simulink model "first"  (R2023b)
settings: Solver=FixedStepAuto  StartTime=0.0  StopTime=10  FixedStep=0.001  RelTol=1e-3
undefined symbols (not defined in the file): A1, A2, B, B2, C2, D2, K1, K2, w0, x0
settings Model: Creator=evdokiiagalkina  LastModifiedBy=evdokiiagalkina

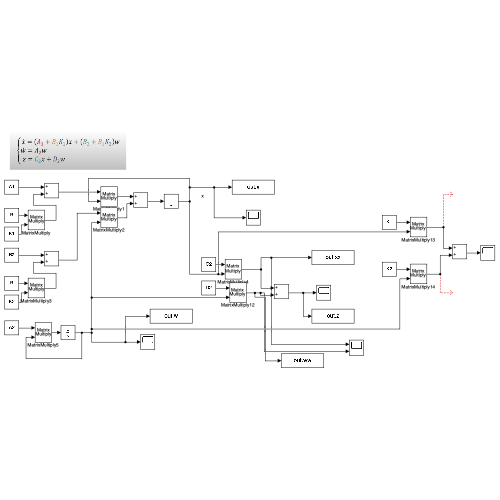
[thumbnail: Simulink's stored preview of the top-level diagram]
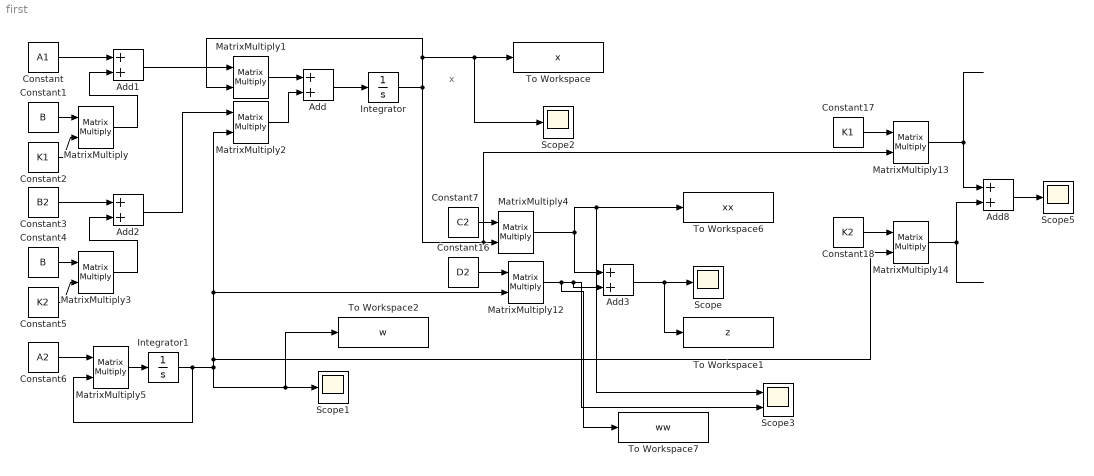
== system first ==
  note: x
  Add{,1..3,8} (5 alike) : Sum
  Constant : Constant  Value=A1  VectorParams1D=off
  Constant1 : Constant  Value=B  VectorParams1D=off
  Constant16 : Constant  Value=D2  VectorParams1D=off
  Constant17 : Constant  Value=K1  VectorParams1D=off
  Constant18 : Constant  Value=K2  VectorParams1D=off
  Constant2 : Constant  Value=K1  VectorParams1D=off
  Constant3 : Constant  Value=B2  VectorParams1D=off
  Constant4 : Constant  Value=B  VectorParams1D=off
  Constant5 : Constant  Value=K2  VectorParams1D=off
  Constant6 : Constant  Value=A2  VectorParams1D=off
  Constant7 : Constant  Value=C2  VectorParams1D=off
  Integrator : Integrator  InitialCondition=x0
  Integrator1 : Integrator  InitialCondition=w0
  MatrixMultiply{,1..5,12..14} (9 alike) : Product  Multiplication=Matrix(*)
  Scope{,1..2,5} (4 alike) : Scope
  Scope3 : Scope  NumInputPorts=2
  To Workspace : ToWorkspace  VariableName=x  SaveFormat=Timeseries  SampleTime=-1
  To Workspace1 : ToWorkspace  VariableName=z  SaveFormat=Timeseries  SampleTime=-1
  To Workspace2 : ToWorkspace  VariableName=w  SaveFormat=Timeseries  SampleTime=-1
  To Workspace6 : ToWorkspace  VariableName=xx  SaveFormat=Timeseries  SampleTime=-1
  To Workspace7 : ToWorkspace  VariableName=ww  SaveFormat=Timeseries  SampleTime=-1
  wires:
  Add/1 -> Integrator/1
  Constant2/1 -> MatrixMultiply/2
  MatrixMultiply1/1 -> Add/1
  MatrixMultiply2/1 -> Add/2
  Constant1/1 -> MatrixMultiply/1
  Constant/1 -> Add1/1
  MatrixMultiply/1 -> Add1/2
  Add1/1 -> MatrixMultiply1/1
  MatrixMultiply3/1 -> Add2/2
  Constant4/1 -> MatrixMultiply3/1
  Constant3/1 -> Add2/1
  Constant5/1 -> MatrixMultiply3/2
  Add2/1 -> MatrixMultiply2/1
  MatrixMultiply5/1 -> Integrator1/1
  Constant6/1 -> MatrixMultiply5/1
  Constant7/1 -> MatrixMultiply4/1
  Integrator/1 -> MatrixMultiply13/2, MatrixMultiply4/2, MatrixMultiply1/2, Scope2/1, To Workspace/1
  MatrixMultiply4/1 -> Add3/1, Scope3/1, To Workspace6/1
  Integrator1/1 -> MatrixMultiply12/2, MatrixMultiply2/2, MatrixMultiply14/2, To Workspace2/1, Scope1/1, MatrixMultiply5/2
  Add3/1 -> To Workspace1/1, Scope/1
  Constant16/1 -> MatrixMultiply12/1
  MatrixMultiply12/1 -> Scope3/2, Add3/2, To Workspace7/1
  Constant17/1 -> MatrixMultiply13/1
  Constant18/1 -> MatrixMultiply14/1
  MatrixMultiply13/1 -> Add8/1
  MatrixMultiply14/1 -> Add8/2
  Add8/1 -> Scope5/1
